simulink model "CAN_Model"  (R2018a)
settings: Solver=VariableStepAuto  StartTime=0.0  StopTime=12.4  RelTol=1e-3
InitFcn:
  | clc;
  | clear;
  | 
  | readyToSend = 1;
libraries: simulink_extras x1
settings Model: Creator=Emiliano  LastModifiedBy=Emiliano

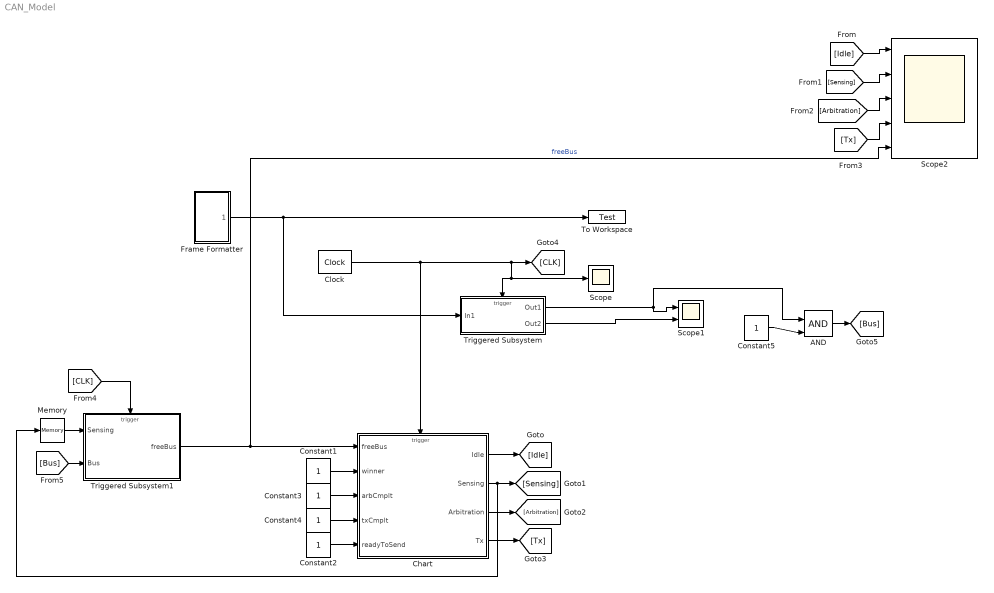
== system CAN_Model ==
  AND : Logic  IconShape=distinctive  AllPortsSameDT=off  OutDataTypeStr=boolean
  Chart : Stateflow chart  TreatAsAtomicUnit=on
  Clock : simulink_extras/Flip Flops/Clock  period=0.2
  Constant{1..5} (5 alike) : Constant
  Frame Formatter : Subsystem
  Memory : Memory  InheritSampleTime=on
  Scope : Scope
  Scope1 : Scope  NumInputPorts=2
  Scope2 : Scope  NumInputPorts=5
  To Workspace : ToWorkspace  VariableName=Test  SaveFormat=Timeseries  SampleTime=-1
  Triggered Subsystem : Subsystem  TreatAsAtomicUnit=on
  Triggered Subsystem1 : Subsystem  TreatAsAtomicUnit=on
  wires:
  Triggered Subsystem/1(Out1) -> Scope1/1, AND/1
  Clock/1 -> Chart/Trigger, [CLK], Triggered Subsystem/Trigger, Scope/1
  Frame Formatter/1(Frame) -> Triggered Subsystem/1(In1), To Workspace/1
  Triggered Subsystem/2(Out2) -> Scope1/2
  Constant1/1 -> Chart/2(winner)
  Constant3/1 -> Chart/3(arbCmplt)
  Constant4/1 -> Chart/4(txCmplt)
  Constant2/1 -> Chart/5(readyToSend)
  Chart/1(" Idle") -> [Idle]
  Chart/3(" Arbitration") -> [Arbitration]
  Chart/4(" Tx") -> [Tx]
  [Idle] -> Scope2/1
  [Sensing] -> Scope2/2
  [Arbitration] -> Scope2/3
  [Tx] -> Scope2/4
  [CLK] -> Triggered Subsystem1/Trigger
  Constant5/1 -> AND/2
  AND/1 -> [Bus]
  [Bus] -> Triggered Subsystem1/2(Bus)
  Triggered Subsystem1/1("freeBus ") -> Chart/1(freeBus), Scope2/5  "freeBus"
  Chart/2(" Sensing") -> Memory/1, [Sensing]
  Memory/1 -> Triggered Subsystem1/1(Sensing)

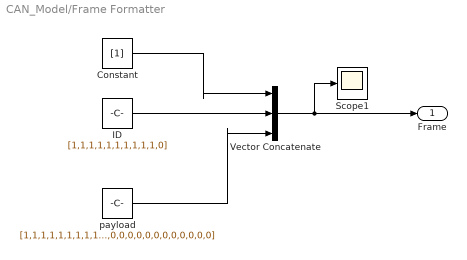
== system CAN_Model/Frame Formatter ==
  Constant : Constant  Value=[1]
  ID : Constant  Value=[1,1,1,1,1,1,1,1,1,1,0]
  Scope1 : Scope
  Vector Concatenate : Concatenate  NumInputs=3
  "payload " : Constant  Value=[1,1,1,1,1,1,1,1,1,1,1,1,1,1,1,1,1,1,1,1,1,1,1,1,1,0,0,0,0,0,0,0,0,0,0,0,0,0,0,0,0,0,0,0,0,0,0,0,0,0]
  Frame : Outport
  wires:
  ID/1 -> Vector Concatenate/2
  Constant/1 -> Vector Concatenate/1
  "payload "/1 -> Vector Concatenate/3
  Vector Concatenate/1 -> Frame/1, Scope1/1

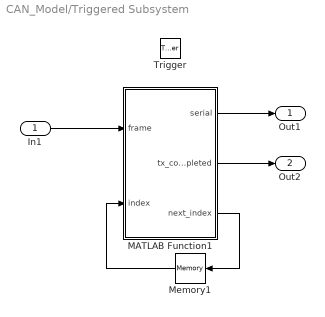
== system CAN_Model/Triggered Subsystem ==
  In1 : Inport
  Trigger : TriggerPort  VariantControl=Variant
  MATLAB Function1 : MATLAB Function  TreatAsAtomicUnit=on
  Memory1 : Memory  InitialCondition=1  InheritSampleTime=on
  Out1 : Outport
  Out2 : Outport  Port=2
  wires:
  In1/1 -> MATLAB Function1/1(frame)
  Memory1/1 -> MATLAB Function1/2(index)
  MATLAB Function1/1(serial) -> Out1/1
  MATLAB Function1/3(next_index) -> Memory1/1
  MATLAB Function1/2(tx_completed) -> Out2/1

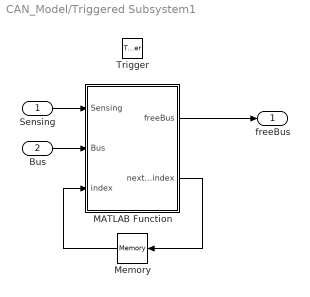
== system CAN_Model/Triggered Subsystem1 ==
  Sensing : Inport
  Bus : Inport  Port=2
  Trigger : TriggerPort  VariantControl=Variant
  MATLAB Function : MATLAB Function  TreatAsAtomicUnit=on
  Memory : Memory  InheritSampleTime=on
  "freeBus " : Outport
  wires:
  Sensing/1 -> MATLAB Function/1(Sensing)
  Bus/1 -> MATLAB Function/2(Bus)
  MATLAB Function/2(next_index) -> Memory/1
  Memory/1 -> MATLAB Function/3(index)
  MATLAB Function/1(freeBus) -> "freeBus "/1

== matlab function CAN_Model/Triggered Subsystem1/MATLAB Function ==
  data: Sensing input; freeBus output; Bus input; index input; next_index output
function [freeBus, next_index] = fcn(Sensing, Bus, index)

freeBus = 0;

if Sensing == 1
    if Bus == 1
        if index < 10
            next_index = index + 1;
        else
            next_index = 0;
            freeBus = 1;
        end
    else
        next_index = 0;
    end
else
   next_index = 0;
end

end

== matlab function CAN_Model/Triggered Subsystem/MATLAB Function1 ==
  data: frame input; serial output; tx_completed output; index input; next_index output
function [serial,  tx_completed ,next_index]  = fcn(frame, index)

frame_size = size(frame);
if index > frame_size
    serial = 0;
    tx_completed = 10;
    next_index = 1;
else
    serial = frame(index);
    next_index = index + 1;
    tx_completed = 0;
end
end

== stateflow chart CAN_Model/Chart ==
  settings: executeAtInitialization=1
  state Idle
  state Sensing
  state Tx
  state Arbitration
  (default) -> Idle
  Idle -> Idle [order 2] : [readyToSend == 0]
  Idle -> Sensing [order 1] : [readyToSend > 0]
  Tx -> Idle [order 1] : [txCmplt == 1]
  Sensing -> Sensing [order 1] : [freeBus == 0]
  Arbitration -> Sensing [order 2] : [winner == 0 && arbCmplt == 1]
  Tx -> Tx [order 2] : [txCmplt == 0]
  Sensing -> Arbitration [order 2] : [freeBus == 1]
  Arbitration -> Tx [order 1] : [winner == 1 && arbCmplt == 1]
  Arbitration -> Arbitration [order 3] : [arbCmplt == 0]
  data: freeBus input; winner input; Idle output boolean; Sensing output boolean; Arbitration output boolean; Tx output boolean; arbCmplt input; txCmplt input; readyToSend input
  events: Start input RISING_EDGE_EVENT
